simulink model "Pokus14_Equality_Comparator"  (Simulink 8.1)
settings: Solver=ode45  StartTime=0.0  StopTime=10.0  RelTol=1e-3
libraries: Arithmetic_Operations_Lib x8, commutil2 x2
settings Model: Creator=uzivatel  LastModifiedBy=uzivatel
settings DataIOCC: SignalLoggingSaveFormat=Dataset
settings OptimizationCC: ExpressionDepthLimit=128
settings DebuggingCC: FcnCallInpInsideContextMsg=EnableAllAsError
settings GRTTargetCC: CombineOutputUpdateFcns=on  GRTInterface=off

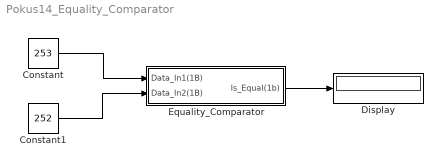
== system Pokus14_Equality_Comparator ==
  Constant : Constant  Value=253
  Constant1 : Constant  Value=252
  Display : Display
  Equality_Comparator : Subsystem
  wires:
  Constant/1 -> Equality_Comparator/1(Data_In1(1B))
  Constant1/1 -> Equality_Comparator/2(Data_In2(1B))
  Equality_Comparator/1(Is_Equal(1b)) -> Display/1

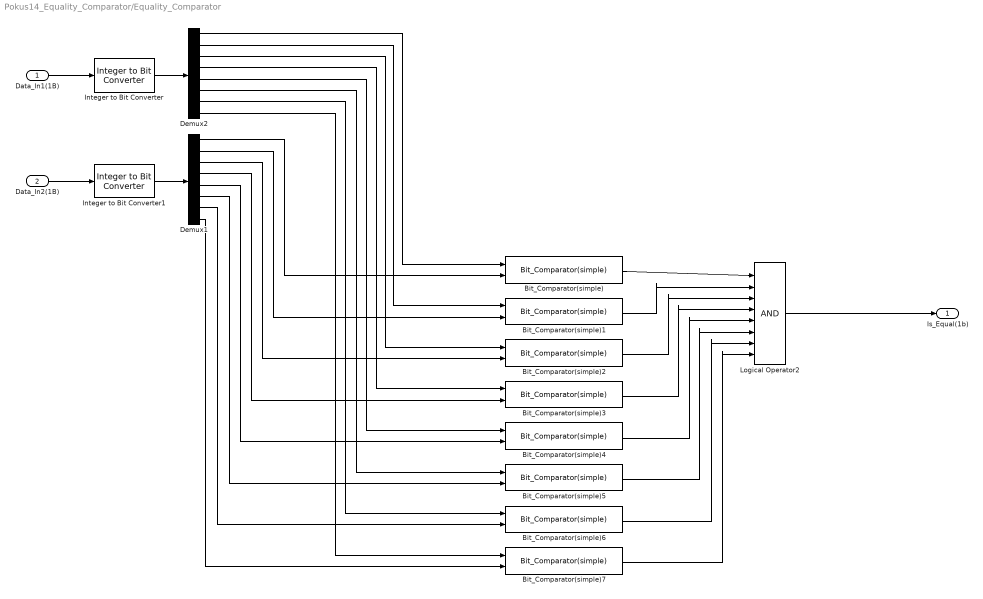
== system Pokus14_Equality_Comparator/Equality_Comparator ==
  Data_In1(1B) : Inport
  Data_In2(1B) : Inport  Port=2
  Bit_Comparator(simple){,1..7} (8 alike) : Arithmetic_Operations_Lib/Arithmetic_Operations_Lib/Bit_Comparator(simple)
  Demux1 : Demux  Outputs=8
  Demux2 : Demux  Outputs=8
  Integer to Bit Converter : commutil2/Integer to Bit Converter  nbits=8  signedInputValues=Unsigned  bitOrder=MSB first  outDtype=boolean
  Integer to Bit Converter1 : commutil2/Integer to Bit Converter  nbits=8  signedInputValues=Unsigned  bitOrder=MSB first  outDtype=boolean
  Logical Operator2 : Logic  Inputs=8  IconShape=distinctive  AllPortsSameDT=off  OutDataTypeStr=boolean
  Is_Equal(1b) : Outport
  wires:
  Integer to Bit Converter/1 -> Demux2/1
  Integer to Bit Converter1/1 -> Demux1/1
  Bit_Comparator(simple)/1 -> Logical Operator2/1
  Bit_Comparator(simple)1/1 -> Logical Operator2/2
  Bit_Comparator(simple)2/1 -> Logical Operator2/3
  Bit_Comparator(simple)3/1 -> Logical Operator2/4
  Bit_Comparator(simple)4/1 -> Logical Operator2/5
  Bit_Comparator(simple)5/1 -> Logical Operator2/6
  Bit_Comparator(simple)6/1 -> Logical Operator2/7
  Bit_Comparator(simple)7/1 -> Logical Operator2/8
  Demux1/8 -> Bit_Comparator(simple)7/2
  Demux1/7 -> Bit_Comparator(simple)6/2
  Demux1/6 -> Bit_Comparator(simple)5/2
  Demux1/5 -> Bit_Comparator(simple)4/2
  Demux1/4 -> Bit_Comparator(simple)3/2
  Demux1/3 -> Bit_Comparator(simple)2/2
  Demux1/2 -> Bit_Comparator(simple)1/2
  Demux1/1 -> Bit_Comparator(simple)/2
  Demux2/8 -> Bit_Comparator(simple)7/1
  Demux2/7 -> Bit_Comparator(simple)6/1
  Demux2/6 -> Bit_Comparator(simple)5/1
  Demux2/5 -> Bit_Comparator(simple)4/1
  Demux2/4 -> Bit_Comparator(simple)3/1
  Demux2/3 -> Bit_Comparator(simple)2/1
  Demux2/2 -> Bit_Comparator(simple)1/1
  Demux2/1 -> Bit_Comparator(simple)/1
  Data_In2(1B)/1 -> Integer to Bit Converter1/1
  Data_In1(1B)/1 -> Integer to Bit Converter/1
  Logical Operator2/1 -> Is_Equal(1b)/1
